simulink model "momentum_dump_test"  (R2016b)
settings: Solver=VariableStepAuto  StartTime=0.0  StopTime=5400  RelTol=1e-3
values from neighbouring files (symbols this model uses):
  fsw_params = init_fsw_params()    [momentum_unload_test_init.m]
undefined symbols (not defined in the file or in its folder): DiscIntNeverNeededParam
libraries: aerolibutil x2, dynamics_lib x2, momentum_dump_lib x1, pd_control_lib x1, mag_vec_LS_lib x1, reaction_wheel_assembly_lib x1, command_processing x1
settings Model: Creator=Taylor  LastModifiedBy=Taylor

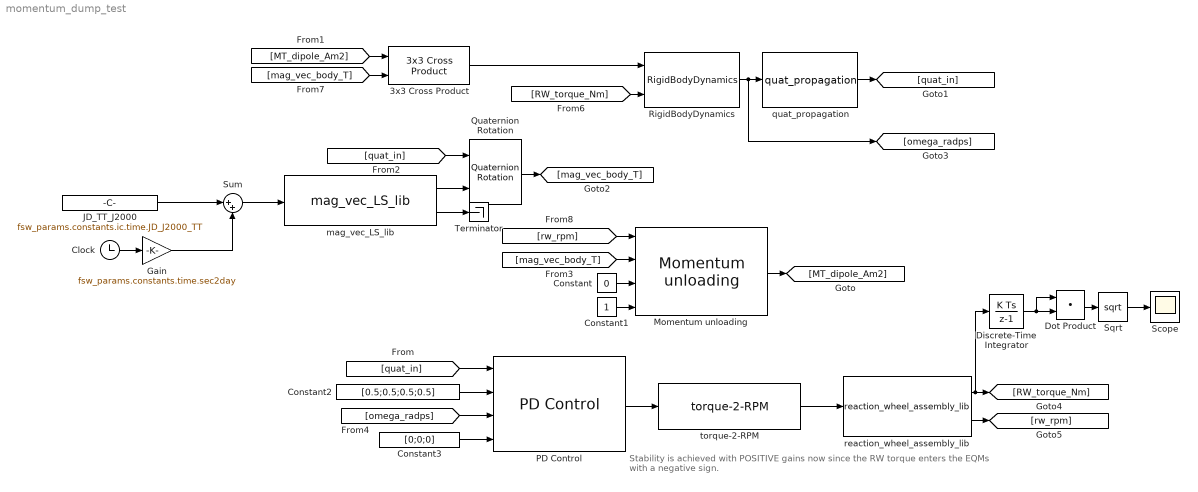
== system momentum_dump_test ==
  note: Stability is achieved with POSITIVE gains now since the RW torque
      | enters the EQMs with a negative sign.
  3x3 Cross Product : aerolibutil/3x3 Cross Product
  Clock : Clock
  Constant : Constant  Value=0
  Constant1 : Constant
  Constant2 : Constant  Value=[0.5;0.5;0.5;0.5]
  Constant3 : Constant  Value=[0;0;0]
  Discrete-Time Integrator : DiscreteIntegrator  InitialConditionSetting=State (most efficient)  SampleTime=-1  ICPrevOutput=DiscIntNeverNeededParam  ICPrevScaledInput=DiscIntNeverNeededParam
  Dot Product : DotProduct  InputSameDT=on  OutDataTypeStr=Inherit: Inherit via internal rule
  Gain : Gain  Gain=fsw_params.constants.time.sec2day
  JD_TT_J2000 : Constant  Value=fsw_params.constants.ic.time.JD_J2000_TT
  Momentum unloading : momentum_dump_lib/Momentum unloading
  PD Control : pd_control_lib/PD Control
  Quaternion Rotation : aerolibutil/Quaternion Rotation
  RigidBodyDynamics : dynamics_lib/Dynamics/RigidBodyDynamics
  Scope : Scope
  Sqrt : Sqrt  SaturateOnIntegerOverflow=on
  Sum : Sum  Inputs=|++
  Terminator : Terminator
  mag_vec_LS_lib : mag_vec_LS_lib/mag_vec_LS_lib
  quat_propagation : dynamics_lib/Dynamics/quat_propagation
  reaction_wheel_assembly_lib : reaction_wheel_assembly_lib/reaction_wheel_assembly_lib
  torque-2-RPM : command_processing/command_processing/torque-2-RPM
  wires:
  3x3 Cross Product/1 -> RigidBodyDynamics/1
  [RW_torque_Nm] -> RigidBodyDynamics/2
  RigidBodyDynamics/1 -> [omega_radps], quat_propagation/1
  [MT_dipole_Am2] -> 3x3 Cross Product/1
  [mag_vec_body_T] -> 3x3 Cross Product/2
  Momentum unloading/1 -> [MT_dipole_Am2]
  [quat_in] -> PD Control/1
  quat_propagation/1 -> [quat_in]
  [quat_in] -> Quaternion Rotation/1
  mag_vec_LS_lib/1 -> Quaternion Rotation/2
  Quaternion Rotation/1 -> [mag_vec_body_T]
  [mag_vec_body_T] -> Momentum unloading/2
  Constant/1 -> Momentum unloading/3
  Constant1/1 -> Momentum unloading/4
  Constant2/1 -> PD Control/2
  Constant3/1 -> PD Control/4
  [omega_radps] -> PD Control/3
  reaction_wheel_assembly_lib/1 -> Discrete-Time Integrator/1, [RW_torque_Nm]
  torque-2-RPM/1 -> reaction_wheel_assembly_lib/1
  reaction_wheel_assembly_lib/2 -> [rw_rpm]
  [rw_rpm] -> Momentum unloading/1
  mag_vec_LS_lib/2 -> Terminator/1
  Clock/1 -> Gain/1
  Gain/1 -> Sum/2
  Sum/1 -> mag_vec_LS_lib/1
  JD_TT_J2000/1 -> Sum/1
  PD Control/1 -> torque-2-RPM/1
  Discrete-Time Integrator/1 -> Dot Product/1, Dot Product/2
  Dot Product/1 -> Sqrt/1
  Sqrt/1 -> Scope/1
